simulink model "WheelModel"  (R2018b)
settings: Solver=VariableStepAuto  StartTime=0.0  StopTime=10.0  RelTol=1e-3
values from neighbouring files (symbols this model uses):
  g = 9.81    [SetCoefficients.m]    (also in SetCoefficients_QC.m)
  kt = 14e4    (= 140000)    [SetCoefficients.m]    (also in SetCoefficients_QC.m)
  m2 = 20    [SetCoefficients.m]    (also in SetCoefficients_QC.m)
undefined symbols (not defined in the file or in its folder): Fs, k
settings Model: Creator=joebe  LastModifiedBy=joebe

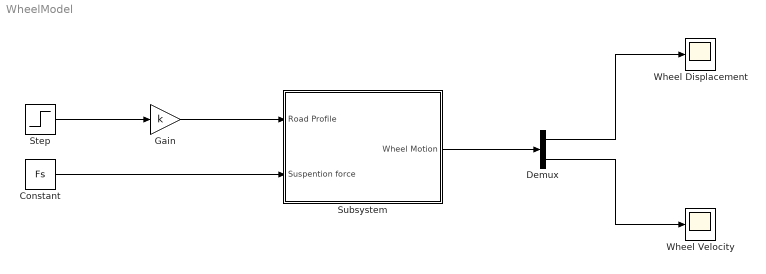
== system WheelModel ==
  Constant : Constant  Value=Fs
  Demux : Demux  Outputs=2
  Gain : Gain  Gain=k
  Step : Step  SampleTime=0
  Subsystem : Subsystem
  Wheel Displacement : Scope
  Wheel Velocity : Scope
  wires:
  Step/1 -> Gain/1
  Subsystem/1(Wheel Motion) -> Demux/1
  Demux/2 -> Wheel Velocity/1
  Demux/1 -> Wheel Displacement/1
  Constant/1 -> Subsystem/2(Suspention force)
  Gain/1 -> Subsystem/1(Road Profile)

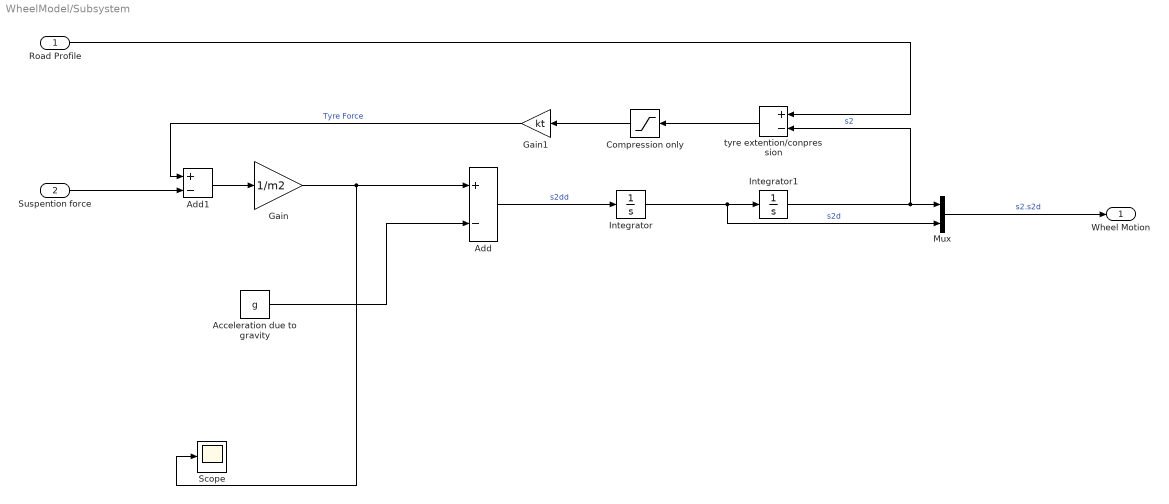
== system WheelModel/Subsystem ==
  Road Profile : Inport
  Suspention force : Inport  Port=2
  Acceleration due to gravity : Constant  Value=g
  Add : Sum  Inputs=+-
  Add1 : Sum  Inputs=+-
  Compression only : Saturate  UpperLimit=100000000000000000000000000000000000000000000  LowerLimit=0  OutMin=0  RndMeth=Nearest
  Gain : Gain  Gain=1/m2
  Gain1 : Gain  Gain=kt
  Integrator : Integrator
  Integrator1 : Integrator
  Mux : Mux  Inputs=2
  Scope : Scope
  tyre extention/conpression : Sum  Inputs=+-
  Wheel Motion : Outport
  wires:
  Gain1/1 -> Add1/1  "Tyre Force"
  Gain/1 -> Scope/1, Add/1
  Suspention force/1 -> Add1/2
  Add/1 -> Integrator/1  "s2dd"
  Acceleration due to gravity/1 -> Add/2
  Integrator1/1 -> tyre extention/conpression/2, Mux/1  "s2"
  Road Profile/1 -> tyre extention/conpression/1
  tyre extention/conpression/1 -> Compression only/1
  Mux/1 -> Wheel Motion/1  "s2.s2d"
  Integrator/1 -> Mux/2, Integrator1/1  "s2d"
  Add1/1 -> Gain/1
  Compression only/1 -> Gain1/1
